simulink model "ES241A_MotAg2Meas"
settings: Solver=FixedStepDiscrete  SolverMode=SingleTasking  StartTime=0.0  StopTime=1  FixedStep=0.002  RelTol=1e-3
values from neighbouring files (symbols this model uses):
  ARCHGLBPRM_2PI_ULS_F32 = DataDict.Constant    [ES241A_MotAg2Meas_DataDict.m]
  FLTINJ_MOTAG2MEAS_MOTAG2MECL = DataDict.Constant    [ES241A_MotAg2Meas_DataDict.m]
  MOTAG2ANSINCOSFLTFAILSTEP_CNT_U16 = DataDict.Constant    [ES241A_MotAg2Meas_DataDict.m]
  MOTAG2ANSINCOSFLTPASSSTEP_CNT_U16 = DataDict.Constant    [ES241A_MotAg2Meas_DataDict.m]
  MotAg2MeasOffs = DataDict.Calibration    [ES241A_MotAg2Meas_DataDict.m]
  MOTAG2MECLMAX_MOTREV_F32 = DataDict.Constant    [ES241A_MotAg2Meas_DataDict.m]
  MOTAG2MECLMIN_MOTREV_F32 = DataDict.Constant    [ES241A_MotAg2Meas_DataDict.m]
  VALMAXERR_VOLTSQD_F32 = DataDict.Constant    [ES241A_MotAg2Meas_DataDict.m]
  VALMINERR_VOLTSQD_F32 = DataDict.Constant    [ES241A_MotAg2Meas_DataDict.m]
undefined symbols (not defined in the file or in its folder): NtcNr1, NtcSts1, sigbuilder_block
libraries: simulink x12, NxtrLim x2, FloatToFixd x1, NxtrMath x1
(part 3 of 3)

== system ES241A_MotAg2Meas/MotAg2Meas/MotAg2MeasPer1/AnalogMsbDiagnostics/RollCnt_Qulfr_Calc/DebounceStepSelection/CopyRight2 ==

== system ES241A_MotAg2Meas/MotAg2Meas/MotAg2MeasPer1/AnalogMsbDiagnostics/RollCnt_Qulfr_Calc/DebounceStepSelection/Debounce_FailStep ==
  Action Port : ActionPort  ActionType=else
  Constant2 : Constant  Value=MOTAG2ANSINCOSFLTFAILSTEP_CNT_U16
  CopyRight2 : Subsystem  Description=|  mask(Copyright Information){none=on}
      | Copyright info block.                                               
      |                                                                     
      | Place copyright information at the top of every subsystem in design.
      mask prompts: none "No parameters"
      mask help: Place copyright information at the top of every subsystem in design.
      mask Display:
      | NxtrConf = 'Nexteer Confidential';
      | 
      | sys = bdroot; %handle for the current model ("system")
      | first = get_param(sys,'Created');
      | if(isempty(first))
      |     first = datestr(now,'yyyy');
      | else
      |     first = first(end-3:end);  %year is last four digits
      | end
      | 
      | last = get_param(sys,'LastModifiedDate');
      | if isempty(last)
      |     last = datestr(now,'yyyy');
      | else
      |     last = last(end-3:end);
      | end
      | 
      | if strcmp(first,last)
      |     fprintf('%s -- Copyright %s Nexteer',NxtrConf,first)
      | else
      |     fprintf('%s -- %s%s- %s Nexteer',NxtrConf,char(169),first,last)
      | end
  Enumerated Constant : simulink/Sources/Enumerated Constant  OutDataTypeStr=Enum: NtcSts1  Value=NtcSts1.NTCSTS_PREFAILD  SampleTime=inf
  NtcSts : Outport
  DebounceStep : Outport  Port=2
  wires:
  Constant2/1 -> DebounceStep/1
  Enumerated Constant/1 -> NtcSts/1

== system ES241A_MotAg2Meas/MotAg2Meas/MotAg2MeasPer1/AnalogMsbDiagnostics/RollCnt_Qulfr_Calc/DebounceStepSelection/Debounce_PassStep ==
  Action Port : ActionPort  ActionType=then
  Constant3 : Constant  Value=MOTAG2ANSINCOSFLTPASSSTEP_CNT_U16
  CopyRight2 : Subsystem  Description=|  mask(Copyright Information){none=on}
      | Copyright info block.                                               
      |                                                                     
      | Place copyright information at the top of every subsystem in design.
      mask prompts: none "No parameters"
      mask help: Place copyright information at the top of every subsystem in design.
      mask Display:
      | NxtrConf = 'Nexteer Confidential';
      | 
      | sys = bdroot; %handle for the current model ("system")
      | first = get_param(sys,'Created');
      | if(isempty(first))
      |     first = datestr(now,'yyyy');
      | else
      |     first = first(end-3:end);  %year is last four digits
      | end
      | 
      | last = get_param(sys,'LastModifiedDate');
      | if isempty(last)
      |     last = datestr(now,'yyyy');
      | else
      |     last = last(end-3:end);
      | end
      | 
      | if strcmp(first,last)
      |     fprintf('%s -- Copyright %s Nexteer',NxtrConf,first)
      | else
      |     fprintf('%s -- %s%s- %s Nexteer',NxtrConf,char(169),first,last)
      | end
  Enumerated Constant : simulink/Sources/Enumerated Constant  OutDataTypeStr=Enum: NtcSts1  Value=NtcSts1.NTCSTS_PREPASSD  SampleTime=inf
  DebounceStep : Outport
  NtcSts : Outport  Port=2
  wires:
  Constant3/1 -> DebounceStep/1
  Enumerated Constant/1 -> NtcSts/1

== system ES241A_MotAg2Meas/MotAg2Meas/MotAg2MeasPer1/AnalogMsbDiagnostics/RollCnt_Qulfr_Calc/GetNtcQlfr/CopyRight2 ==

== system ES241A_MotAg2Meas/MotAg2Meas/MotAg2MeasPer1/AnalogMsbDiagnostics/RollCnt_Qulfr_Calc/SetNtcSts/CopyRight2 ==

== system ES241A_MotAg2Meas/MotAg2Meas/MotAg2MeasPer1/AnalogMsbDiagnostics/TestFail/If Action Subsystem/CopyRight2 ==

== system ES241A_MotAg2Meas/MotAg2Meas/MotAg2MeasPer1/AnalogMsbDiagnostics/TestFail/If Action Subsystem1/CopyRight2 ==

== system ES241A_MotAg2Meas/MotAg2Meas/MotAg2MeasPer1/AnalogMsbDiagnostics/TestFail/If Action Subsystem2/CopyRight2 ==

== system ES241A_MotAg2Meas/MotAg2Meas/MotAg2MeasPer1/AnalogMsbDiagnostics/TestFail/If Action Subsystem3/CopyRight2 ==

== system ES241A_MotAg2Meas/MotAg2Meas/MotAg2MeasPer1/AnalogMsbDiagnostics/TestFail/Normal/CopyRight2 ==

== system ES241A_MotAg2Meas/MotAg2Meas/MotAg2MeasPer1/AnalogMsbDiagnostics/TestFail/SinCosMaxError/CopyRight2 ==

== system ES241A_MotAg2Meas/MotAg2Meas/MotAg2MeasPer1/AnalogMsbDiagnostics/TestFail/SinCosMinError/CopyRight2 ==

== system ES241A_MotAg2Meas/MotAg2Meas/MotAg2MeasPer1/MotPos_ArcTan/MotAg2MeclMeas/NegativePolarity/CopyRight2 ==

== system ES241A_MotAg2Meas/MotAg2Meas/MotAg2MeasPer1/MotPos_ArcTan/MotAg2MeclMeas/PositivePolarity/CopyRight2 ==

== system ES241A_MotAg2Meas/MotAg2Meas/MotAg2MeasPer1/AnalogMsbDiagnostics/RollCnt_Qulfr_Calc/DebounceStepSelection/Debounce_FailStep/CopyRight2 ==

== system ES241A_MotAg2Meas/MotAg2Meas/MotAg2MeasPer1/AnalogMsbDiagnostics/RollCnt_Qulfr_Calc/DebounceStepSelection/Debounce_PassStep/CopyRight2 ==

== stateflow chart ES241A_MotAg2Meas/MotAg2Meas/MotAg2MeasPer1/MotPos_ArcTan/LimitMotAg2Meas/NormalizeMotAg2Mecl ==
  (default) -> (junction 3)
  (junction 3) -> (junction 5) : {MotAg2MeclVar=MotAg2MeclIn;}
  (junction 5) -> (junction 7) [order 2] : [MotAg2MeclVar<0]
  (junction 5) -> (junction 6) [order 1] : [MotAg2MeclVar>1]
  (junction 6) -> (junction 5) : {MotAg2MeclVar=MotAg2MeclVar-1;}
  (junction 7) -> (junction 5) : {MotAg2MeclVar=MotAg2MeclVar+1;}
  (junction 5) -> (junction 13) [order 3] : {MotAg2Mecl=MotAg2MeclVar;}
  data: MotAg2MeclIn input; MotAg2Mecl output single; MotAg2MeclVar local single

== stateflow chart ES241A_MotAg2Meas/MotAg2Meas/MotAg2MeasPer1/AnalogMsbDiagnostics/RollCnt_Qulfr_Calc/RollingCntr_Calc ==
  settings: stateMachineType=MEALY_MACHINE
  (default) -> (junction 4)
  (junction 4) -> (junction 6) [order 1] : [TestOk==1]
  (junction 6) -> (junction 36) [order 2] : {RollgCntr = PrevRollgCntr+1;}
  (junction 4) -> (junction 20) [order 2]
  (junction 6) -> (junction 36) [order 1] : [PrevRollgCntr == 255]
      | {
      | RollgCntr = 0;
      | }
  (junction 36) -> (junction 20)
  data: TestOk input; PrevRollgCntr input uint8 [0..255] =0; RollgCntr output uint8

== stateflow chart ES241A_MotAg2Meas/MotAg2Meas/MotAg2MeasPer1/AnalogMsbDiagnostics/RollCnt_Qulfr_Calc/SetNtcSts/ISO Fault Debounce Design ==
  note: NTCSTS_PASSD           (0)
      | NTCSTS_FAILD             (1)
      | NTCSTS_PREPASSD   (2)
      | NTCSTS_PREFAILD     (3)
      |
      | SIGQLFR_NORES        (0)
      | SIGQLFR_PASSD         (1)
      | SIGQLFR_FAILD           (2)
  note: Pass Loop
  note: Fail Loop
  note: 
  (default) -> (junction 89)
  (junction 89) -> (junction 95) [order 1] : [NtcSts ==3]
  (junction 89) -> (junction 93) [order 2] : [NtcSts ==2]
  (junction 89) -> (junction 141) [order 3] : [NtcSts ==1]
      | { ErrAcc = 32767;
      | Qualifier =2;
      |  }
  (junction 89) -> (junction 141) [order 4] : [NtcSts ==0]
      | { ErrAcc = -32768;
      | Qualifier=1;
      | }
  (junction 95) -> (junction 111) [order 1] : [ErrAcc <=0]
      | {ErrAcc = DebStep;}
  (junction 95) -> (junction 103) [order 2]
  (junction 93) -> (junction 123) [order 2] : {
      | ErrAcc = ErrAcc - DebStep;
      | }
  (junction 93) -> (junction 123) [order 1] : [(ErrAcc - DebStep) <= -32768]
      | {
      | ErrAcc = -32768;
      | Qualifier=1;
      | }
  (junction 103) -> (junction 111) [order 1] : [(ErrAcc + DebStep) <32767]
      | {ErrAcc = ErrAcc + DebStep;}
  (junction 103) -> (junction 111) [order 2] : {ErrAcc = 32767;
      | Qualifier =2;}
  (junction 123) -> (junction 141)
  (junction 111) -> (junction 141)
  (junction 141) -> (junction 159) [order 2] : {ErrAcc = 0;
      | Qualifier =0;
      | }
  (junction 141) -> (junction 159) [order 1] : [SvcClr ==0]
  data: NtcSts input uint8; Qualifier output uint8; DebStep input uint16; ErrAcc local int16; SvcClr input
